simulink model "LQR_obs_noise"  (R2025b)
settings: Solver=VariableStepAuto  StartTime=0.0  StopTime=50  RelTol=1e-3
values from neighbouring files (symbols this model uses):
  a = -log(OS/100)    [pole_placement_ctrl.m]
  A = [0 1 0 0;     (m_b*g*r^2)/(I_b*l) 0 (m_b*g*r^2)/(I_b) 0 ;      0 0 0 1;    20 0 (M_r*d*g)/I_r 0 ]    [Copy_of_LQR_ctrl.m]    (also in LQR_ctrl.m = [0 1 0 0;     A1(1,1) 0 A1(1,2) 0;     0 0 0 1;     A1(2,1) ; Rlocus_ctrl.m = [0 1 0 0;     A1(1,1) 0 A1(1,2) 0;     0 0 0 1;     A1(2,1) ; State4.m = [0 1 0 0;     A1(1,1) 0 A1(1,2) 0;     0 0 0 1;     A1(2,1) ; pole_placement_ctrl.m = [0 1 0 0;     A1(1,1) 0 0 0;     0 0 0 1;    A1(2,1) 0 A1(2,)
  B = -[0 ; 0; 0 ; ((I_w/R) + (M_w+M_r)*R)/(I_r)]    [Copy_of_LQR_ctrl.m]    (also in LQR_ctrl.m = -[0 ; B1(1); 0 ; B1(2)]; Rlocus_ctrl.m = -[0 ; B1(1); 0 ; B1(2)]; State4.m = -[0 ; B1(1); 0 ; B1(2)]; pole_placement_ctrl.m = -[0 ; B1(1); 0 ; B1(2)])
  C = [0 0 1 0]    [Copy_of_LQR_ctrl.m]    (also in LQR_ctrl.m; Rlocus_ctrl.m = eye(4); State4.m = eye(4); pole_placement_ctrl.m)
  K = lqr(A, B, Q, R)    [State4.m]    (also in pole_placement_ctrl.m = place(A,B,poles))
  Ke = L    [Copy_of_LQR_ctrl.m]    (also in LQR_ctrl.m)
  x0 = [0.01, 0, deg2rad(5),0]'    [Copy_of_LQR_ctrl.m]    (also in LQR_ctrl.m; State4.m = x0 - x_ref; pole_placement_ctrl.m = [0.005, 0, deg2rad(0.2),0]')
  x0_o = [0.02;0;deg2rad(7.5);0]    [Copy_of_LQR_ctrl.m]    (also in LQR_ctrl.m = [0.025;0;deg2rad(5.25);0])
undefined symbols (not defined in the file or in its folder): b, dspblkCoreblockFVToolHelper, gcbh
libraries: simulink x1
settings Model: Creator=Abhi  LastModifiedBy=Abhi

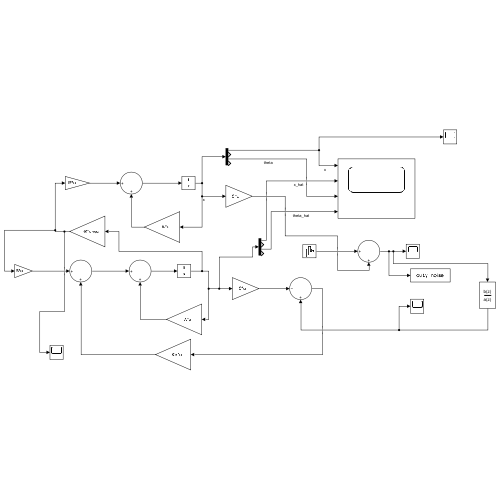
[thumbnail: Simulink's stored preview of the top-level diagram]
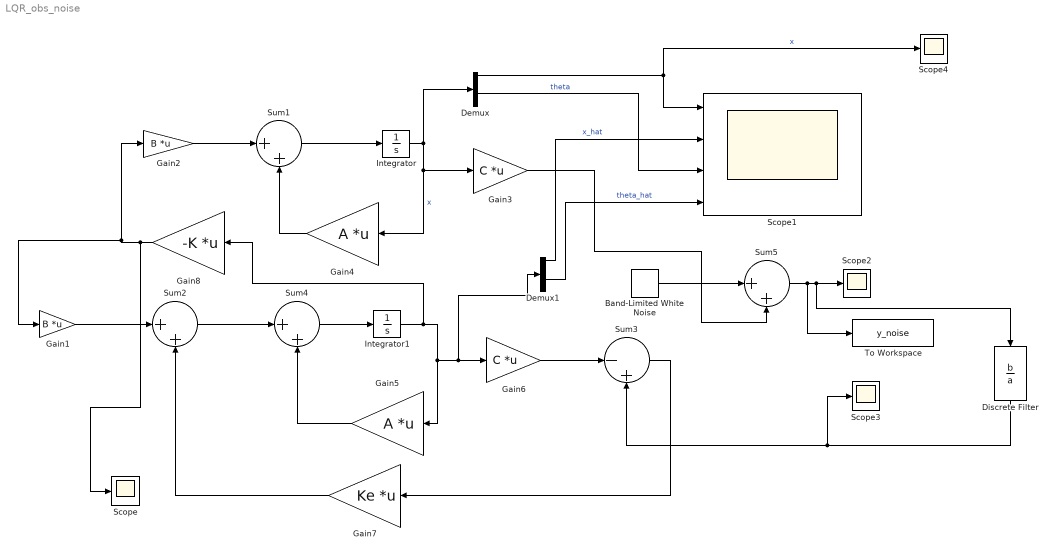
== system LQR_obs_noise ==
  Band-Limited White Noise : simulink/Sources/Band-Limited White Noise  Cov=[0.00000000001]  Ts=0.00001  seed=[23341]
  Demux : Demux
  Demux1 : Demux
  Discrete Filter : DiscreteFilter  LoadFcn=dspblkCoreblockFVToolHelper(gcbh,'load');  Numerator=b  Denominator=a
      settings: CopyFcn=dspblkCoreblockFVToolHelper(gcbh,'copy');  DeleteFcn=dspblkCoreblockFVToolHelper(gcbh,'close');  ModelCloseFcn=dspblkCoreblockFVToolHelper(gcbh,'close');  PreSaveFcn=dspblkCoreblockFVToolHelper(gcbh,'presave');  PostSaveFcn=dspblkCoreblockFVToolHelper(gcbh,'postsave');  CloseFcn=dspblkCoreblockFVToolHelper(gcbh,'close');
  Gain1 : Gain  Gain=B  Multiplication=Matrix(K*u)
  Gain2 : Gain  Gain=B  Multiplication=Matrix(K*u)
  Gain3 : Gain  Gain=C  Multiplication=Matrix(K*u)
  Gain4 : Gain  Gain=A  Multiplication=Matrix(K*u)
  Gain5 : Gain  Gain=A  Multiplication=Matrix(K*u)
  Gain6 : Gain  Gain=C  Multiplication=Matrix(K*u)
  Gain7 : Gain  Gain=Ke  Multiplication=Matrix(K*u)
  Gain8 : Gain  Gain=-K  Multiplication=Matrix(K*u) (u vector)
  Integrator : Integrator  InitialCondition=x0
  Integrator1 : Integrator  InitialCondition=x0_o
  Scope{,2..4} (4 alike) : Scope
      Scope settings: SampleTime=1e-4  ActiveDisplayYMinimum=-3.4028150972495675E+6  ActiveDisplayYMaximum=5.6797007294752859E+6
      Scope2 settings: SampleTime=1e-4  ActiveDisplayYMinimum=-0.066239294401067544  ActiveDisplayYMaximum=0.12395772369607108  DataLoggingVariableName=ScopeData2
      Scope3 settings: ActiveDisplayYMinimum=-0.045080883939710548  ActiveDisplayYMaximum=0.1056086210481581  DataLoggingVariableName=ScopeData3
      Scope4 settings: SampleTime=1e-4  ActiveDisplayYMinimum=-0.012681214243520488  ActiveDisplayYMaximum=0.01252013491594672  DataLoggingVariableName=ScopeData4
  Scope1 : Scope  NumInputPorts=4
      settings: SampleTime=1e-4  ActiveDisplayYMinimum=-0.012585123017231463  ActiveDisplayYMaximum=0.012509458113025718
  Sum{1..2,4..5} (4 alike) : Sum  Inputs=|++
  Sum3 : Sum  Inputs=|-+
  To Workspace : ToWorkspace  VariableName=y_noise  SaveFormat=Structure With Time  SampleTime=1e-4
  wires:
  Sum1/1 -> Integrator/1
  Gain3/1 -> Sum5/2
  Gain4/1 -> Sum1/2
  Gain2/1 -> Sum1/1
  Gain1/1 -> Sum2/1
  Integrator/1 -> Gain3/1, Gain4/1, Demux/1  "x"
  Sum3/1 -> Gain7/1
  Integrator1/1 -> Gain8/1, Demux1/1, Gain6/1, Gain5/1
  Gain6/1 -> Sum3/1
  Gain5/1 -> Sum4/2
  Sum2/1 -> Sum4/1
  Sum4/1 -> Integrator1/1
  Gain7/1 -> Sum2/2
  Gain8/1 -> Scope/1, Gain1/1, Gain2/1
  Demux1/1 -> Scope1/2  "x_hat"
  Demux1/3 -> Scope1/4  "theta_hat"
  Demux/3 -> Scope1/3  "theta"
  Demux/1 -> Scope1/1, Scope4/1  "x"
  Band-Limited White Noise/1 -> Sum5/1
  Sum5/1 -> Discrete Filter/1, Scope2/1, To Workspace/1
  Discrete Filter/1 -> Scope3/1, Sum3/2
